simulink model "pipelined_and_spatial_parallelism"  (R2015b)
settings: Solver=FixedStepDiscrete  SolverMode=SingleTasking  StartTime=0.0  StopTime=5e-4  RelTol=1e-3
undefined symbols (not defined in the file): a, b
libraries: shlslibv1 x5277
(part 19 of 23)

== system pipelined_and_spatial_parallelism/Simon_encrypt 3/Key_expansion_function2 ==
  k_ii : Inport
  k_ii1 : Inport  Port=2
  k_ii2 : Inport  Port=3
  k_ii3 : Inport  Port=4
  c : Inport  Port=5
  z : Inport  Port=6
  Binary Logic{1..5} (5 alike) : shlslibv1/Math Functions/Binary Logic  syn_binlog_exp=a^b  synBlockType=primitive  synLatency=0  synBlockId=13
  Binary Logic6 : shlslibv1/Math Functions/Binary Logic  syn_binlog_exp=a|b  synBlockType=primitive  synLatency=0  synBlockId=13
  Binary Logic7 : shlslibv1/Math Functions/Binary Logic  syn_binlog_exp=a|b  synBlockType=primitive  synLatency=0  synBlockId=13
  Constant : shlslibv1/Sources/Constant  syn_cst_val=3  syn_cst_format=Specify  syn_cst_wl=4  syn_cst_fl=0  syn_cst_dt=unsigned  syn_cst_rnd=on  syn_cst_st=-1  synBlockType=primitive  synLatency=0  synBlockId=15
  Constant1 : shlslibv1/Sources/Constant  syn_cst_val=1  syn_cst_format=Specify  syn_cst_wl=4  syn_cst_fl=0  syn_cst_dt=unsigned  syn_cst_rnd=on  syn_cst_st=-1  synBlockType=primitive  synLatency=0  synBlockId=15
  Constant2 : shlslibv1/Sources/Constant  syn_cst_val=13  syn_cst_format=Specify  syn_cst_wl=4  syn_cst_fl=0  syn_cst_dt=unsigned  syn_cst_rnd=on  syn_cst_st=-1  synBlockType=primitive  synLatency=0  synBlockId=15
  Constant3 : shlslibv1/Sources/Constant  syn_cst_val=15  syn_cst_format=Specify  syn_cst_wl=4  syn_cst_fl=0  syn_cst_dt=unsigned  syn_cst_rnd=on  syn_cst_st=-1  synBlockType=primitive  synLatency=0  synBlockId=15
  Shifter : shlslibv1/Math Functions/Shifter  syn_shifter_opr=<<  syn_out_f=Automatic  syn_out_wl=16  syn_out_fl=8  syn_out_dt=signed  synBlockType=primitive  synLatency=0  synBlockId=12
  Shifter1 : shlslibv1/Math Functions/Shifter  syn_shifter_opr=>>  syn_out_f=Automatic  syn_out_wl=16  syn_out_fl=8  syn_out_dt=signed  synBlockType=primitive  synLatency=0  synBlockId=12
  Shifter2 : shlslibv1/Math Functions/Shifter  syn_shifter_opr=>>  syn_out_f=Automatic  syn_out_wl=16  syn_out_fl=8  syn_out_dt=signed  synBlockType=primitive  synLatency=0  synBlockId=12
  Shifter3 : shlslibv1/Math Functions/Shifter  syn_shifter_opr=<<  syn_out_f=Automatic  syn_out_wl=16  syn_out_fl=8  syn_out_dt=signed  synBlockType=primitive  synLatency=0  synBlockId=12
  K_iii : Outport
  Kiii1 : Outport  Port=2
  Kiii2 : Outport  Port=3
  Kiii3 : Outport  Port=4
  wires:
  Binary Logic1/1 -> Shifter3/1, Shifter2/1, Binary Logic3/2
  Constant/1 -> Shifter1/2
  Constant1/1 -> Shifter2/2
  Binary Logic2/1 -> Kiii3/1
  Binary Logic4/1 -> Binary Logic2/1
  k_ii/1 -> Binary Logic3/1
  k_ii1/1 -> K_iii/1, Binary Logic1/1
  z/1 -> Binary Logic5/1
  c/1 -> Binary Logic5/2
  k_ii2/1 -> Kiii1/1
  k_ii3/1 -> Shifter/1, Shifter1/1, Kiii2/1
  Binary Logic3/1 -> Binary Logic4/1
  Binary Logic5/1 -> Binary Logic2/2
  Constant2/1 -> Shifter/2
  Shifter1/1 -> Binary Logic6/1
  Shifter/1 -> Binary Logic6/2
  Binary Logic6/1 -> Binary Logic1/2
  Constant3/1 -> Shifter3/2
  Shifter2/1 -> Binary Logic7/1
  Shifter3/1 -> Binary Logic7/2
  Binary Logic7/1 -> Binary Logic4/2

== system pipelined_and_spatial_parallelism/Simon_encrypt 3/Key_expansion_function20 ==
  k_ii : Inport
  k_ii1 : Inport  Port=2
  k_ii2 : Inport  Port=3
  k_ii3 : Inport  Port=4
  c : Inport  Port=5
  z : Inport  Port=6
  Binary Logic{1..5} (5 alike) : shlslibv1/Math Functions/Binary Logic  syn_binlog_exp=a^b  synBlockType=primitive  synLatency=0  synBlockId=13
  Binary Logic6 : shlslibv1/Math Functions/Binary Logic  syn_binlog_exp=a|b  synBlockType=primitive  synLatency=0  synBlockId=13
  Binary Logic7 : shlslibv1/Math Functions/Binary Logic  syn_binlog_exp=a|b  synBlockType=primitive  synLatency=0  synBlockId=13
  Constant : shlslibv1/Sources/Constant  syn_cst_val=3  syn_cst_format=Specify  syn_cst_wl=4  syn_cst_fl=0  syn_cst_dt=unsigned  syn_cst_rnd=on  syn_cst_st=-1  synBlockType=primitive  synLatency=0  synBlockId=15
  Constant1 : shlslibv1/Sources/Constant  syn_cst_val=1  syn_cst_format=Specify  syn_cst_wl=4  syn_cst_fl=0  syn_cst_dt=unsigned  syn_cst_rnd=on  syn_cst_st=-1  synBlockType=primitive  synLatency=0  synBlockId=15
  Constant2 : shlslibv1/Sources/Constant  syn_cst_val=13  syn_cst_format=Specify  syn_cst_wl=4  syn_cst_fl=0  syn_cst_dt=unsigned  syn_cst_rnd=on  syn_cst_st=-1  synBlockType=primitive  synLatency=0  synBlockId=15
  Constant3 : shlslibv1/Sources/Constant  syn_cst_val=15  syn_cst_format=Specify  syn_cst_wl=4  syn_cst_fl=0  syn_cst_dt=unsigned  syn_cst_rnd=on  syn_cst_st=-1  synBlockType=primitive  synLatency=0  synBlockId=15
  Shifter : shlslibv1/Math Functions/Shifter  syn_shifter_opr=<<  syn_out_f=Automatic  syn_out_wl=16  syn_out_fl=8  syn_out_dt=signed  synBlockType=primitive  synLatency=0  synBlockId=12
  Shifter1 : shlslibv1/Math Functions/Shifter  syn_shifter_opr=>>  syn_out_f=Automatic  syn_out_wl=16  syn_out_fl=8  syn_out_dt=signed  synBlockType=primitive  synLatency=0  synBlockId=12
  Shifter2 : shlslibv1/Math Functions/Shifter  syn_shifter_opr=>>  syn_out_f=Automatic  syn_out_wl=16  syn_out_fl=8  syn_out_dt=signed  synBlockType=primitive  synLatency=0  synBlockId=12
  Shifter3 : shlslibv1/Math Functions/Shifter  syn_shifter_opr=<<  syn_out_f=Automatic  syn_out_wl=16  syn_out_fl=8  syn_out_dt=signed  synBlockType=primitive  synLatency=0  synBlockId=12
  K_iii : Outport
  Kiii1 : Outport  Port=2
  Kiii2 : Outport  Port=3
  Kiii3 : Outport  Port=4
  wires:
  Binary Logic1/1 -> Shifter3/1, Shifter2/1, Binary Logic3/2
  Constant/1 -> Shifter1/2
  Constant1/1 -> Shifter2/2
  Binary Logic2/1 -> Kiii3/1
  Binary Logic4/1 -> Binary Logic2/1
  k_ii/1 -> Binary Logic3/1
  k_ii1/1 -> K_iii/1, Binary Logic1/1
  z/1 -> Binary Logic5/1
  c/1 -> Binary Logic5/2
  k_ii2/1 -> Kiii1/1
  k_ii3/1 -> Shifter/1, Shifter1/1, Kiii2/1
  Binary Logic3/1 -> Binary Logic4/1
  Binary Logic5/1 -> Binary Logic2/2
  Constant2/1 -> Shifter/2
  Shifter1/1 -> Binary Logic6/1
  Shifter/1 -> Binary Logic6/2
  Binary Logic6/1 -> Binary Logic1/2
  Constant3/1 -> Shifter3/2
  Shifter2/1 -> Binary Logic7/1
  Shifter3/1 -> Binary Logic7/2
  Binary Logic7/1 -> Binary Logic4/2

== system pipelined_and_spatial_parallelism/Simon_encrypt 3/Key_expansion_function21 ==
  k_ii : Inport
  k_ii1 : Inport  Port=2
  k_ii2 : Inport  Port=3
  k_ii3 : Inport  Port=4
  c : Inport  Port=5
  z : Inport  Port=6
  Binary Logic{1..5} (5 alike) : shlslibv1/Math Functions/Binary Logic  syn_binlog_exp=a^b  synBlockType=primitive  synLatency=0  synBlockId=13
  Binary Logic6 : shlslibv1/Math Functions/Binary Logic  syn_binlog_exp=a|b  synBlockType=primitive  synLatency=0  synBlockId=13
  Binary Logic7 : shlslibv1/Math Functions/Binary Logic  syn_binlog_exp=a|b  synBlockType=primitive  synLatency=0  synBlockId=13
  Constant : shlslibv1/Sources/Constant  syn_cst_val=3  syn_cst_format=Specify  syn_cst_wl=4  syn_cst_fl=0  syn_cst_dt=unsigned  syn_cst_rnd=on  syn_cst_st=-1  synBlockType=primitive  synLatency=0  synBlockId=15
  Constant1 : shlslibv1/Sources/Constant  syn_cst_val=1  syn_cst_format=Specify  syn_cst_wl=4  syn_cst_fl=0  syn_cst_dt=unsigned  syn_cst_rnd=on  syn_cst_st=-1  synBlockType=primitive  synLatency=0  synBlockId=15
  Constant2 : shlslibv1/Sources/Constant  syn_cst_val=13  syn_cst_format=Specify  syn_cst_wl=4  syn_cst_fl=0  syn_cst_dt=unsigned  syn_cst_rnd=on  syn_cst_st=-1  synBlockType=primitive  synLatency=0  synBlockId=15
  Constant3 : shlslibv1/Sources/Constant  syn_cst_val=15  syn_cst_format=Specify  syn_cst_wl=4  syn_cst_fl=0  syn_cst_dt=unsigned  syn_cst_rnd=on  syn_cst_st=-1  synBlockType=primitive  synLatency=0  synBlockId=15
  Shifter : shlslibv1/Math Functions/Shifter  syn_shifter_opr=<<  syn_out_f=Automatic  syn_out_wl=16  syn_out_fl=8  syn_out_dt=signed  synBlockType=primitive  synLatency=0  synBlockId=12
  Shifter1 : shlslibv1/Math Functions/Shifter  syn_shifter_opr=>>  syn_out_f=Automatic  syn_out_wl=16  syn_out_fl=8  syn_out_dt=signed  synBlockType=primitive  synLatency=0  synBlockId=12
  Shifter2 : shlslibv1/Math Functions/Shifter  syn_shifter_opr=>>  syn_out_f=Automatic  syn_out_wl=16  syn_out_fl=8  syn_out_dt=signed  synBlockType=primitive  synLatency=0  synBlockId=12
  Shifter3 : shlslibv1/Math Functions/Shifter  syn_shifter_opr=<<  syn_out_f=Automatic  syn_out_wl=16  syn_out_fl=8  syn_out_dt=signed  synBlockType=primitive  synLatency=0  synBlockId=12
  K_iii : Outport
  Kiii1 : Outport  Port=2
  Kiii2 : Outport  Port=3
  Kiii3 : Outport  Port=4
  wires:
  Binary Logic1/1 -> Shifter3/1, Shifter2/1, Binary Logic3/2
  Constant/1 -> Shifter1/2
  Constant1/1 -> Shifter2/2
  Binary Logic2/1 -> Kiii3/1
  Binary Logic4/1 -> Binary Logic2/1
  k_ii/1 -> Binary Logic3/1
  k_ii1/1 -> K_iii/1, Binary Logic1/1
  z/1 -> Binary Logic5/1
  c/1 -> Binary Logic5/2
  k_ii2/1 -> Kiii1/1
  k_ii3/1 -> Shifter/1, Shifter1/1, Kiii2/1
  Binary Logic3/1 -> Binary Logic4/1
  Binary Logic5/1 -> Binary Logic2/2
  Constant2/1 -> Shifter/2
  Shifter1/1 -> Binary Logic6/1
  Shifter/1 -> Binary Logic6/2
  Binary Logic6/1 -> Binary Logic1/2
  Constant3/1 -> Shifter3/2
  Shifter2/1 -> Binary Logic7/1
  Shifter3/1 -> Binary Logic7/2
  Binary Logic7/1 -> Binary Logic4/2

== system pipelined_and_spatial_parallelism/Simon_encrypt 3/Key_expansion_function22 ==
  k_ii : Inport
  k_ii1 : Inport  Port=2
  k_ii2 : Inport  Port=3
  k_ii3 : Inport  Port=4
  c : Inport  Port=5
  z : Inport  Port=6
  Binary Logic{1..5} (5 alike) : shlslibv1/Math Functions/Binary Logic  syn_binlog_exp=a^b  synBlockType=primitive  synLatency=0  synBlockId=13
  Binary Logic6 : shlslibv1/Math Functions/Binary Logic  syn_binlog_exp=a|b  synBlockType=primitive  synLatency=0  synBlockId=13
  Binary Logic7 : shlslibv1/Math Functions/Binary Logic  syn_binlog_exp=a|b  synBlockType=primitive  synLatency=0  synBlockId=13
  Constant : shlslibv1/Sources/Constant  syn_cst_val=3  syn_cst_format=Specify  syn_cst_wl=4  syn_cst_fl=0  syn_cst_dt=unsigned  syn_cst_rnd=on  syn_cst_st=-1  synBlockType=primitive  synLatency=0  synBlockId=15
  Constant1 : shlslibv1/Sources/Constant  syn_cst_val=1  syn_cst_format=Specify  syn_cst_wl=4  syn_cst_fl=0  syn_cst_dt=unsigned  syn_cst_rnd=on  syn_cst_st=-1  synBlockType=primitive  synLatency=0  synBlockId=15
  Constant2 : shlslibv1/Sources/Constant  syn_cst_val=13  syn_cst_format=Specify  syn_cst_wl=4  syn_cst_fl=0  syn_cst_dt=unsigned  syn_cst_rnd=on  syn_cst_st=-1  synBlockType=primitive  synLatency=0  synBlockId=15
  Constant3 : shlslibv1/Sources/Constant  syn_cst_val=15  syn_cst_format=Specify  syn_cst_wl=4  syn_cst_fl=0  syn_cst_dt=unsigned  syn_cst_rnd=on  syn_cst_st=-1  synBlockType=primitive  synLatency=0  synBlockId=15
  Shifter : shlslibv1/Math Functions/Shifter  syn_shifter_opr=<<  syn_out_f=Automatic  syn_out_wl=16  syn_out_fl=8  syn_out_dt=signed  synBlockType=primitive  synLatency=0  synBlockId=12
  Shifter1 : shlslibv1/Math Functions/Shifter  syn_shifter_opr=>>  syn_out_f=Automatic  syn_out_wl=16  syn_out_fl=8  syn_out_dt=signed  synBlockType=primitive  synLatency=0  synBlockId=12
  Shifter2 : shlslibv1/Math Functions/Shifter  syn_shifter_opr=>>  syn_out_f=Automatic  syn_out_wl=16  syn_out_fl=8  syn_out_dt=signed  synBlockType=primitive  synLatency=0  synBlockId=12
  Shifter3 : shlslibv1/Math Functions/Shifter  syn_shifter_opr=<<  syn_out_f=Automatic  syn_out_wl=16  syn_out_fl=8  syn_out_dt=signed  synBlockType=primitive  synLatency=0  synBlockId=12
  K_iii : Outport
  Kiii1 : Outport  Port=2
  Kiii2 : Outport  Port=3
  Kiii3 : Outport  Port=4
  wires:
  Binary Logic1/1 -> Shifter3/1, Shifter2/1, Binary Logic3/2
  Constant/1 -> Shifter1/2
  Constant1/1 -> Shifter2/2
  Binary Logic2/1 -> Kiii3/1
  Binary Logic4/1 -> Binary Logic2/1
  k_ii/1 -> Binary Logic3/1
  k_ii1/1 -> K_iii/1, Binary Logic1/1
  z/1 -> Binary Logic5/1
  c/1 -> Binary Logic5/2
  k_ii2/1 -> Kiii1/1
  k_ii3/1 -> Shifter/1, Shifter1/1, Kiii2/1
  Binary Logic3/1 -> Binary Logic4/1
  Binary Logic5/1 -> Binary Logic2/2
  Constant2/1 -> Shifter/2
  Shifter1/1 -> Binary Logic6/1
  Shifter/1 -> Binary Logic6/2
  Binary Logic6/1 -> Binary Logic1/2
  Constant3/1 -> Shifter3/2
  Shifter2/1 -> Binary Logic7/1
  Shifter3/1 -> Binary Logic7/2
  Binary Logic7/1 -> Binary Logic4/2

== system pipelined_and_spatial_parallelism/Simon_encrypt 3/Key_expansion_function23 ==
  k_ii : Inport
  k_ii1 : Inport  Port=2
  k_ii2 : Inport  Port=3
  k_ii3 : Inport  Port=4
  c : Inport  Port=5
  z : Inport  Port=6
  Binary Logic{1..5} (5 alike) : shlslibv1/Math Functions/Binary Logic  syn_binlog_exp=a^b  synBlockType=primitive  synLatency=0  synBlockId=13
  Binary Logic6 : shlslibv1/Math Functions/Binary Logic  syn_binlog_exp=a|b  synBlockType=primitive  synLatency=0  synBlockId=13
  Binary Logic7 : shlslibv1/Math Functions/Binary Logic  syn_binlog_exp=a|b  synBlockType=primitive  synLatency=0  synBlockId=13
  Constant : shlslibv1/Sources/Constant  syn_cst_val=3  syn_cst_format=Specify  syn_cst_wl=4  syn_cst_fl=0  syn_cst_dt=unsigned  syn_cst_rnd=on  syn_cst_st=-1  synBlockType=primitive  synLatency=0  synBlockId=15
  Constant1 : shlslibv1/Sources/Constant  syn_cst_val=1  syn_cst_format=Specify  syn_cst_wl=4  syn_cst_fl=0  syn_cst_dt=unsigned  syn_cst_rnd=on  syn_cst_st=-1  synBlockType=primitive  synLatency=0  synBlockId=15
  Constant2 : shlslibv1/Sources/Constant  syn_cst_val=13  syn_cst_format=Specify  syn_cst_wl=4  syn_cst_fl=0  syn_cst_dt=unsigned  syn_cst_rnd=on  syn_cst_st=-1  synBlockType=primitive  synLatency=0  synBlockId=15
  Constant3 : shlslibv1/Sources/Constant  syn_cst_val=15  syn_cst_format=Specify  syn_cst_wl=4  syn_cst_fl=0  syn_cst_dt=unsigned  syn_cst_rnd=on  syn_cst_st=-1  synBlockType=primitive  synLatency=0  synBlockId=15
  Shifter : shlslibv1/Math Functions/Shifter  syn_shifter_opr=<<  syn_out_f=Automatic  syn_out_wl=16  syn_out_fl=8  syn_out_dt=signed  synBlockType=primitive  synLatency=0  synBlockId=12
  Shifter1 : shlslibv1/Math Functions/Shifter  syn_shifter_opr=>>  syn_out_f=Automatic  syn_out_wl=16  syn_out_fl=8  syn_out_dt=signed  synBlockType=primitive  synLatency=0  synBlockId=12
  Shifter2 : shlslibv1/Math Functions/Shifter  syn_shifter_opr=>>  syn_out_f=Automatic  syn_out_wl=16  syn_out_fl=8  syn_out_dt=signed  synBlockType=primitive  synLatency=0  synBlockId=12
  Shifter3 : shlslibv1/Math Functions/Shifter  syn_shifter_opr=<<  syn_out_f=Automatic  syn_out_wl=16  syn_out_fl=8  syn_out_dt=signed  synBlockType=primitive  synLatency=0  synBlockId=12
  K_iii : Outport
  Kiii1 : Outport  Port=2
  Kiii2 : Outport  Port=3
  Kiii3 : Outport  Port=4
  wires:
  Binary Logic1/1 -> Shifter3/1, Shifter2/1, Binary Logic3/2
  Constant/1 -> Shifter1/2
  Constant1/1 -> Shifter2/2
  Binary Logic2/1 -> Kiii3/1
  Binary Logic4/1 -> Binary Logic2/1
  k_ii/1 -> Binary Logic3/1
  k_ii1/1 -> K_iii/1, Binary Logic1/1
  z/1 -> Binary Logic5/1
  c/1 -> Binary Logic5/2
  k_ii2/1 -> Kiii1/1
  k_ii3/1 -> Shifter/1, Shifter1/1, Kiii2/1
  Binary Logic3/1 -> Binary Logic4/1
  Binary Logic5/1 -> Binary Logic2/2
  Constant2/1 -> Shifter/2
  Shifter1/1 -> Binary Logic6/1
  Shifter/1 -> Binary Logic6/2
  Binary Logic6/1 -> Binary Logic1/2
  Constant3/1 -> Shifter3/2
  Shifter2/1 -> Binary Logic7/1
  Shifter3/1 -> Binary Logic7/2
  Binary Logic7/1 -> Binary Logic4/2

== system pipelined_and_spatial_parallelism/Simon_encrypt 3/Key_expansion_function24 ==
  k_ii : Inport
  k_ii1 : Inport  Port=2
  k_ii2 : Inport  Port=3
  k_ii3 : Inport  Port=4
  c : Inport  Port=5
  z : Inport  Port=6
  Binary Logic{1..5} (5 alike) : shlslibv1/Math Functions/Binary Logic  syn_binlog_exp=a^b  synBlockType=primitive  synLatency=0  synBlockId=13
  Binary Logic6 : shlslibv1/Math Functions/Binary Logic  syn_binlog_exp=a|b  synBlockType=primitive  synLatency=0  synBlockId=13
  Binary Logic7 : shlslibv1/Math Functions/Binary Logic  syn_binlog_exp=a|b  synBlockType=primitive  synLatency=0  synBlockId=13
  Constant : shlslibv1/Sources/Constant  syn_cst_val=3  syn_cst_format=Specify  syn_cst_wl=4  syn_cst_fl=0  syn_cst_dt=unsigned  syn_cst_rnd=on  syn_cst_st=-1  synBlockType=primitive  synLatency=0  synBlockId=15
  Constant1 : shlslibv1/Sources/Constant  syn_cst_val=1  syn_cst_format=Specify  syn_cst_wl=4  syn_cst_fl=0  syn_cst_dt=unsigned  syn_cst_rnd=on  syn_cst_st=-1  synBlockType=primitive  synLatency=0  synBlockId=15
  Constant2 : shlslibv1/Sources/Constant  syn_cst_val=13  syn_cst_format=Specify  syn_cst_wl=4  syn_cst_fl=0  syn_cst_dt=unsigned  syn_cst_rnd=on  syn_cst_st=-1  synBlockType=primitive  synLatency=0  synBlockId=15
  Constant3 : shlslibv1/Sources/Constant  syn_cst_val=15  syn_cst_format=Specify  syn_cst_wl=4  syn_cst_fl=0  syn_cst_dt=unsigned  syn_cst_rnd=on  syn_cst_st=-1  synBlockType=primitive  synLatency=0  synBlockId=15
  Shifter : shlslibv1/Math Functions/Shifter  syn_shifter_opr=<<  syn_out_f=Automatic  syn_out_wl=16  syn_out_fl=8  syn_out_dt=signed  synBlockType=primitive  synLatency=0  synBlockId=12
  Shifter1 : shlslibv1/Math Functions/Shifter  syn_shifter_opr=>>  syn_out_f=Automatic  syn_out_wl=16  syn_out_fl=8  syn_out_dt=signed  synBlockType=primitive  synLatency=0  synBlockId=12
  Shifter2 : shlslibv1/Math Functions/Shifter  syn_shifter_opr=>>  syn_out_f=Automatic  syn_out_wl=16  syn_out_fl=8  syn_out_dt=signed  synBlockType=primitive  synLatency=0  synBlockId=12
  Shifter3 : shlslibv1/Math Functions/Shifter  syn_shifter_opr=<<  syn_out_f=Automatic  syn_out_wl=16  syn_out_fl=8  syn_out_dt=signed  synBlockType=primitive  synLatency=0  synBlockId=12
  K_iii : Outport
  Kiii1 : Outport  Port=2
  Kiii2 : Outport  Port=3
  Kiii3 : Outport  Port=4
  wires:
  Binary Logic1/1 -> Shifter3/1, Shifter2/1, Binary Logic3/2
  Constant/1 -> Shifter1/2
  Constant1/1 -> Shifter2/2
  Binary Logic2/1 -> Kiii3/1
  Binary Logic4/1 -> Binary Logic2/1
  k_ii/1 -> Binary Logic3/1
  k_ii1/1 -> K_iii/1, Binary Logic1/1
  z/1 -> Binary Logic5/1
  c/1 -> Binary Logic5/2
  k_ii2/1 -> Kiii1/1
  k_ii3/1 -> Shifter/1, Shifter1/1, Kiii2/1
  Binary Logic3/1 -> Binary Logic4/1
  Binary Logic5/1 -> Binary Logic2/2
  Constant2/1 -> Shifter/2
  Shifter1/1 -> Binary Logic6/1
  Shifter/1 -> Binary Logic6/2
  Binary Logic6/1 -> Binary Logic1/2
  Constant3/1 -> Shifter3/2
  Shifter2/1 -> Binary Logic7/1
  Shifter3/1 -> Binary Logic7/2
  Binary Logic7/1 -> Binary Logic4/2

== system pipelined_and_spatial_parallelism/Simon_encrypt 3/Key_expansion_function25 ==
  k_ii : Inport
  k_ii1 : Inport  Port=2
  k_ii2 : Inport  Port=3
  k_ii3 : Inport  Port=4
  c : Inport  Port=5
  z : Inport  Port=6
  Binary Logic{1..5} (5 alike) : shlslibv1/Math Functions/Binary Logic  syn_binlog_exp=a^b  synBlockType=primitive  synLatency=0  synBlockId=13
  Binary Logic6 : shlslibv1/Math Functions/Binary Logic  syn_binlog_exp=a|b  synBlockType=primitive  synLatency=0  synBlockId=13
  Binary Logic7 : shlslibv1/Math Functions/Binary Logic  syn_binlog_exp=a|b  synBlockType=primitive  synLatency=0  synBlockId=13
  Constant : shlslibv1/Sources/Constant  syn_cst_val=3  syn_cst_format=Specify  syn_cst_wl=4  syn_cst_fl=0  syn_cst_dt=unsigned  syn_cst_rnd=on  syn_cst_st=-1  synBlockType=primitive  synLatency=0  synBlockId=15
  Constant1 : shlslibv1/Sources/Constant  syn_cst_val=1  syn_cst_format=Specify  syn_cst_wl=4  syn_cst_fl=0  syn_cst_dt=unsigned  syn_cst_rnd=on  syn_cst_st=-1  synBlockType=primitive  synLatency=0  synBlockId=15
  Constant2 : shlslibv1/Sources/Constant  syn_cst_val=13  syn_cst_format=Specify  syn_cst_wl=4  syn_cst_fl=0  syn_cst_dt=unsigned  syn_cst_rnd=on  syn_cst_st=-1  synBlockType=primitive  synLatency=0  synBlockId=15
  Constant3 : shlslibv1/Sources/Constant  syn_cst_val=15  syn_cst_format=Specify  syn_cst_wl=4  syn_cst_fl=0  syn_cst_dt=unsigned  syn_cst_rnd=on  syn_cst_st=-1  synBlockType=primitive  synLatency=0  synBlockId=15
  Shifter : shlslibv1/Math Functions/Shifter  syn_shifter_opr=<<  syn_out_f=Automatic  syn_out_wl=16  syn_out_fl=8  syn_out_dt=signed  synBlockType=primitive  synLatency=0  synBlockId=12
  Shifter1 : shlslibv1/Math Functions/Shifter  syn_shifter_opr=>>  syn_out_f=Automatic  syn_out_wl=16  syn_out_fl=8  syn_out_dt=signed  synBlockType=primitive  synLatency=0  synBlockId=12
  Shifter2 : shlslibv1/Math Functions/Shifter  syn_shifter_opr=>>  syn_out_f=Automatic  syn_out_wl=16  syn_out_fl=8  syn_out_dt=signed  synBlockType=primitive  synLatency=0  synBlockId=12
  Shifter3 : shlslibv1/Math Functions/Shifter  syn_shifter_opr=<<  syn_out_f=Automatic  syn_out_wl=16  syn_out_fl=8  syn_out_dt=signed  synBlockType=primitive  synLatency=0  synBlockId=12
  K_iii : Outport
  Kiii1 : Outport  Port=2
  Kiii2 : Outport  Port=3
  Kiii3 : Outport  Port=4
  wires:
  Binary Logic1/1 -> Shifter3/1, Shifter2/1, Binary Logic3/2
  Constant/1 -> Shifter1/2
  Constant1/1 -> Shifter2/2
  Binary Logic2/1 -> Kiii3/1
  Binary Logic4/1 -> Binary Logic2/1
  k_ii/1 -> Binary Logic3/1
  k_ii1/1 -> K_iii/1, Binary Logic1/1
  z/1 -> Binary Logic5/1
  c/1 -> Binary Logic5/2
  k_ii2/1 -> Kiii1/1
  k_ii3/1 -> Shifter/1, Shifter1/1, Kiii2/1
  Binary Logic3/1 -> Binary Logic4/1
  Binary Logic5/1 -> Binary Logic2/2
  Constant2/1 -> Shifter/2
  Shifter1/1 -> Binary Logic6/1
  Shifter/1 -> Binary Logic6/2
  Binary Logic6/1 -> Binary Logic1/2
  Constant3/1 -> Shifter3/2
  Shifter2/1 -> Binary Logic7/1
  Shifter3/1 -> Binary Logic7/2
  Binary Logic7/1 -> Binary Logic4/2

== system pipelined_and_spatial_parallelism/Simon_encrypt 3/Key_expansion_function26 ==
  k_ii : Inport
  k_ii1 : Inport  Port=2
  k_ii2 : Inport  Port=3
  k_ii3 : Inport  Port=4
  c : Inport  Port=5
  z : Inport  Port=6
  Binary Logic{1..5} (5 alike) : shlslibv1/Math Functions/Binary Logic  syn_binlog_exp=a^b  synBlockType=primitive  synLatency=0  synBlockId=13
  Binary Logic6 : shlslibv1/Math Functions/Binary Logic  syn_binlog_exp=a|b  synBlockType=primitive  synLatency=0  synBlockId=13
  Binary Logic7 : shlslibv1/Math Functions/Binary Logic  syn_binlog_exp=a|b  synBlockType=primitive  synLatency=0  synBlockId=13
  Constant : shlslibv1/Sources/Constant  syn_cst_val=3  syn_cst_format=Specify  syn_cst_wl=4  syn_cst_fl=0  syn_cst_dt=unsigned  syn_cst_rnd=on  syn_cst_st=-1  synBlockType=primitive  synLatency=0  synBlockId=15
  Constant1 : shlslibv1/Sources/Constant  syn_cst_val=1  syn_cst_format=Specify  syn_cst_wl=4  syn_cst_fl=0  syn_cst_dt=unsigned  syn_cst_rnd=on  syn_cst_st=-1  synBlockType=primitive  synLatency=0  synBlockId=15
  Constant2 : shlslibv1/Sources/Constant  syn_cst_val=13  syn_cst_format=Specify  syn_cst_wl=4  syn_cst_fl=0  syn_cst_dt=unsigned  syn_cst_rnd=on  syn_cst_st=-1  synBlockType=primitive  synLatency=0  synBlockId=15
  Constant3 : shlslibv1/Sources/Constant  syn_cst_val=15  syn_cst_format=Specify  syn_cst_wl=4  syn_cst_fl=0  syn_cst_dt=unsigned  syn_cst_rnd=on  syn_cst_st=-1  synBlockType=primitive  synLatency=0  synBlockId=15
  Shifter : shlslibv1/Math Functions/Shifter  syn_shifter_opr=<<  syn_out_f=Automatic  syn_out_wl=16  syn_out_fl=8  syn_out_dt=signed  synBlockType=primitive  synLatency=0  synBlockId=12
  Shifter1 : shlslibv1/Math Functions/Shifter  syn_shifter_opr=>>  syn_out_f=Automatic  syn_out_wl=16  syn_out_fl=8  syn_out_dt=signed  synBlockType=primitive  synLatency=0  synBlockId=12
  Shifter2 : shlslibv1/Math Functions/Shifter  syn_shifter_opr=>>  syn_out_f=Automatic  syn_out_wl=16  syn_out_fl=8  syn_out_dt=signed  synBlockType=primitive  synLatency=0  synBlockId=12
  Shifter3 : shlslibv1/Math Functions/Shifter  syn_shifter_opr=<<  syn_out_f=Automatic  syn_out_wl=16  syn_out_fl=8  syn_out_dt=signed  synBlockType=primitive  synLatency=0  synBlockId=12
  K_iii : Outport
  Kiii1 : Outport  Port=2
  Kiii2 : Outport  Port=3
  Kiii3 : Outport  Port=4
  wires:
  Binary Logic1/1 -> Shifter3/1, Shifter2/1, Binary Logic3/2
  Constant/1 -> Shifter1/2
  Constant1/1 -> Shifter2/2
  Binary Logic2/1 -> Kiii3/1
  Binary Logic4/1 -> Binary Logic2/1
  k_ii/1 -> Binary Logic3/1
  k_ii1/1 -> K_iii/1, Binary Logic1/1
  z/1 -> Binary Logic5/1
  c/1 -> Binary Logic5/2
  k_ii2/1 -> Kiii1/1
  k_ii3/1 -> Shifter/1, Shifter1/1, Kiii2/1
  Binary Logic3/1 -> Binary Logic4/1
  Binary Logic5/1 -> Binary Logic2/2
  Constant2/1 -> Shifter/2
  Shifter1/1 -> Binary Logic6/1
  Shifter/1 -> Binary Logic6/2
  Binary Logic6/1 -> Binary Logic1/2
  Constant3/1 -> Shifter3/2
  Shifter2/1 -> Binary Logic7/1
  Shifter3/1 -> Binary Logic7/2
  Binary Logic7/1 -> Binary Logic4/2

== system pipelined_and_spatial_parallelism/Simon_encrypt 3/Key_expansion_function27 ==
  k_ii : Inport
  k_ii1 : Inport  Port=2
  k_ii2 : Inport  Port=3
  k_ii3 : Inport  Port=4
  c : Inport  Port=5
  z : Inport  Port=6
  Binary Logic{1..5} (5 alike) : shlslibv1/Math Functions/Binary Logic  syn_binlog_exp=a^b  synBlockType=primitive  synLatency=0  synBlockId=13
  Binary Logic6 : shlslibv1/Math Functions/Binary Logic  syn_binlog_exp=a|b  synBlockType=primitive  synLatency=0  synBlockId=13
  Binary Logic7 : shlslibv1/Math Functions/Binary Logic  syn_binlog_exp=a|b  synBlockType=primitive  synLatency=0  synBlockId=13
  Constant : shlslibv1/Sources/Constant  syn_cst_val=3  syn_cst_format=Specify  syn_cst_wl=4  syn_cst_fl=0  syn_cst_dt=unsigned  syn_cst_rnd=on  syn_cst_st=-1  synBlockType=primitive  synLatency=0  synBlockId=15
  Constant1 : shlslibv1/Sources/Constant  syn_cst_val=1  syn_cst_format=Specify  syn_cst_wl=4  syn_cst_fl=0  syn_cst_dt=unsigned  syn_cst_rnd=on  syn_cst_st=-1  synBlockType=primitive  synLatency=0  synBlockId=15
  Constant2 : shlslibv1/Sources/Constant  syn_cst_val=13  syn_cst_format=Specify  syn_cst_wl=4  syn_cst_fl=0  syn_cst_dt=unsigned  syn_cst_rnd=on  syn_cst_st=-1  synBlockType=primitive  synLatency=0  synBlockId=15
  Constant3 : shlslibv1/Sources/Constant  syn_cst_val=15  syn_cst_format=Specify  syn_cst_wl=4  syn_cst_fl=0  syn_cst_dt=unsigned  syn_cst_rnd=on  syn_cst_st=-1  synBlockType=primitive  synLatency=0  synBlockId=15
  Shifter : shlslibv1/Math Functions/Shifter  syn_shifter_opr=<<  syn_out_f=Automatic  syn_out_wl=16  syn_out_fl=8  syn_out_dt=signed  synBlockType=primitive  synLatency=0  synBlockId=12
  Shifter1 : shlslibv1/Math Functions/Shifter  syn_shifter_opr=>>  syn_out_f=Automatic  syn_out_wl=16  syn_out_fl=8  syn_out_dt=signed  synBlockType=primitive  synLatency=0  synBlockId=12
  Shifter2 : shlslibv1/Math Functions/Shifter  syn_shifter_opr=>>  syn_out_f=Automatic  syn_out_wl=16  syn_out_fl=8  syn_out_dt=signed  synBlockType=primitive  synLatency=0  synBlockId=12
  Shifter3 : shlslibv1/Math Functions/Shifter  syn_shifter_opr=<<  syn_out_f=Automatic  syn_out_wl=16  syn_out_fl=8  syn_out_dt=signed  synBlockType=primitive  synLatency=0  synBlockId=12
  K_iii : Outport
  Kiii1 : Outport  Port=2
  Kiii2 : Outport  Port=3
  Kiii3 : Outport  Port=4
  wires:
  Binary Logic1/1 -> Shifter3/1, Shifter2/1, Binary Logic3/2
  Constant/1 -> Shifter1/2
  Constant1/1 -> Shifter2/2
  Binary Logic2/1 -> Kiii3/1
  Binary Logic4/1 -> Binary Logic2/1
  k_ii/1 -> Binary Logic3/1
  k_ii1/1 -> K_iii/1, Binary Logic1/1
  z/1 -> Binary Logic5/1
  c/1 -> Binary Logic5/2
  k_ii2/1 -> Kiii1/1
  k_ii3/1 -> Shifter/1, Shifter1/1, Kiii2/1
  Binary Logic3/1 -> Binary Logic4/1
  Binary Logic5/1 -> Binary Logic2/2
  Constant2/1 -> Shifter/2
  Shifter1/1 -> Binary Logic6/1
  Shifter/1 -> Binary Logic6/2
  Binary Logic6/1 -> Binary Logic1/2
  Constant3/1 -> Shifter3/2
  Shifter2/1 -> Binary Logic7/1
  Shifter3/1 -> Binary Logic7/2
  Binary Logic7/1 -> Binary Logic4/2

== system pipelined_and_spatial_parallelism/Simon_encrypt 3/Key_expansion_function29 ==
  k_ii : Inport
  k_ii1 : Inport  Port=2
  k_ii2 : Inport  Port=3
  k_ii3 : Inport  Port=4
  c : Inport  Port=5
  z : Inport  Port=6
  Binary Logic{1..5} (5 alike) : shlslibv1/Math Functions/Binary Logic  syn_binlog_exp=a^b  synBlockType=primitive  synLatency=0  synBlockId=13
  Binary Logic6 : shlslibv1/Math Functions/Binary Logic  syn_binlog_exp=a|b  synBlockType=primitive  synLatency=0  synBlockId=13
  Binary Logic7 : shlslibv1/Math Functions/Binary Logic  syn_binlog_exp=a|b  synBlockType=primitive  synLatency=0  synBlockId=13
  Constant : shlslibv1/Sources/Constant  syn_cst_val=3  syn_cst_format=Specify  syn_cst_wl=4  syn_cst_fl=0  syn_cst_dt=unsigned  syn_cst_rnd=on  syn_cst_st=-1  synBlockType=primitive  synLatency=0  synBlockId=15
  Constant1 : shlslibv1/Sources/Constant  syn_cst_val=1  syn_cst_format=Specify  syn_cst_wl=4  syn_cst_fl=0  syn_cst_dt=unsigned  syn_cst_rnd=on  syn_cst_st=-1  synBlockType=primitive  synLatency=0  synBlockId=15
  Constant2 : shlslibv1/Sources/Constant  syn_cst_val=13  syn_cst_format=Specify  syn_cst_wl=4  syn_cst_fl=0  syn_cst_dt=unsigned  syn_cst_rnd=on  syn_cst_st=-1  synBlockType=primitive  synLatency=0  synBlockId=15
  Constant3 : shlslibv1/Sources/Constant  syn_cst_val=15  syn_cst_format=Specify  syn_cst_wl=4  syn_cst_fl=0  syn_cst_dt=unsigned  syn_cst_rnd=on  syn_cst_st=-1  synBlockType=primitive  synLatency=0  synBlockId=15
  Shifter : shlslibv1/Math Functions/Shifter  syn_shifter_opr=<<  syn_out_f=Automatic  syn_out_wl=16  syn_out_fl=8  syn_out_dt=signed  synBlockType=primitive  synLatency=0  synBlockId=12
  Shifter1 : shlslibv1/Math Functions/Shifter  syn_shifter_opr=>>  syn_out_f=Automatic  syn_out_wl=16  syn_out_fl=8  syn_out_dt=signed  synBlockType=primitive  synLatency=0  synBlockId=12
  Shifter2 : shlslibv1/Math Functions/Shifter  syn_shifter_opr=>>  syn_out_f=Automatic  syn_out_wl=16  syn_out_fl=8  syn_out_dt=signed  synBlockType=primitive  synLatency=0  synBlockId=12
  Shifter3 : shlslibv1/Math Functions/Shifter  syn_shifter_opr=<<  syn_out_f=Automatic  syn_out_wl=16  syn_out_fl=8  syn_out_dt=signed  synBlockType=primitive  synLatency=0  synBlockId=12
  K_iii : Outport
  Kiii1 : Outport  Port=2
  Kiii2 : Outport  Port=3
  Kiii3 : Outport  Port=4
  wires:
  Binary Logic1/1 -> Shifter3/1, Shifter2/1, Binary Logic3/2
  Constant/1 -> Shifter1/2
  Constant1/1 -> Shifter2/2
  Binary Logic2/1 -> Kiii3/1
  Binary Logic4/1 -> Binary Logic2/1
  k_ii/1 -> Binary Logic3/1
  k_ii1/1 -> K_iii/1, Binary Logic1/1
  z/1 -> Binary Logic5/1
  c/1 -> Binary Logic5/2
  k_ii2/1 -> Kiii1/1
  k_ii3/1 -> Shifter/1, Shifter1/1, Kiii2/1
  Binary Logic3/1 -> Binary Logic4/1
  Binary Logic5/1 -> Binary Logic2/2
  Constant2/1 -> Shifter/2
  Shifter1/1 -> Binary Logic6/1
  Shifter/1 -> Binary Logic6/2
  Binary Logic6/1 -> Binary Logic1/2
  Constant3/1 -> Shifter3/2
  Shifter2/1 -> Binary Logic7/1
  Shifter3/1 -> Binary Logic7/2
  Binary Logic7/1 -> Binary Logic4/2

== system pipelined_and_spatial_parallelism/Simon_encrypt 3/Key_expansion_function3 ==
  k_ii : Inport
  k_ii1 : Inport  Port=2
  k_ii2 : Inport  Port=3
  k_ii3 : Inport  Port=4
  c : Inport  Port=5
  z : Inport  Port=6
  Binary Logic{1..5} (5 alike) : shlslibv1/Math Functions/Binary Logic  syn_binlog_exp=a^b  synBlockType=primitive  synLatency=0  synBlockId=13
  Binary Logic6 : shlslibv1/Math Functions/Binary Logic  syn_binlog_exp=a|b  synBlockType=primitive  synLatency=0  synBlockId=13
  Binary Logic7 : shlslibv1/Math Functions/Binary Logic  syn_binlog_exp=a|b  synBlockType=primitive  synLatency=0  synBlockId=13
  Constant : shlslibv1/Sources/Constant  syn_cst_val=3  syn_cst_format=Specify  syn_cst_wl=4  syn_cst_fl=0  syn_cst_dt=unsigned  syn_cst_rnd=on  syn_cst_st=-1  synBlockType=primitive  synLatency=0  synBlockId=15
  Constant1 : shlslibv1/Sources/Constant  syn_cst_val=1  syn_cst_format=Specify  syn_cst_wl=4  syn_cst_fl=0  syn_cst_dt=unsigned  syn_cst_rnd=on  syn_cst_st=-1  synBlockType=primitive  synLatency=0  synBlockId=15
  Constant2 : shlslibv1/Sources/Constant  syn_cst_val=13  syn_cst_format=Specify  syn_cst_wl=4  syn_cst_fl=0  syn_cst_dt=unsigned  syn_cst_rnd=on  syn_cst_st=-1  synBlockType=primitive  synLatency=0  synBlockId=15
  Constant3 : shlslibv1/Sources/Constant  syn_cst_val=15  syn_cst_format=Specify  syn_cst_wl=4  syn_cst_fl=0  syn_cst_dt=unsigned  syn_cst_rnd=on  syn_cst_st=-1  synBlockType=primitive  synLatency=0  synBlockId=15
  Shifter : shlslibv1/Math Functions/Shifter  syn_shifter_opr=<<  syn_out_f=Automatic  syn_out_wl=16  syn_out_fl=8  syn_out_dt=signed  synBlockType=primitive  synLatency=0  synBlockId=12
  Shifter1 : shlslibv1/Math Functions/Shifter  syn_shifter_opr=>>  syn_out_f=Automatic  syn_out_wl=16  syn_out_fl=8  syn_out_dt=signed  synBlockType=primitive  synLatency=0  synBlockId=12
  Shifter2 : shlslibv1/Math Functions/Shifter  syn_shifter_opr=>>  syn_out_f=Automatic  syn_out_wl=16  syn_out_fl=8  syn_out_dt=signed  synBlockType=primitive  synLatency=0  synBlockId=12
  Shifter3 : shlslibv1/Math Functions/Shifter  syn_shifter_opr=<<  syn_out_f=Automatic  syn_out_wl=16  syn_out_fl=8  syn_out_dt=signed  synBlockType=primitive  synLatency=0  synBlockId=12
  K_iii : Outport
  Kiii1 : Outport  Port=2
  Kiii2 : Outport  Port=3
  Kiii3 : Outport  Port=4
  wires:
  Binary Logic1/1 -> Shifter3/1, Shifter2/1, Binary Logic3/2
  Constant/1 -> Shifter1/2
  Constant1/1 -> Shifter2/2
  Binary Logic2/1 -> Kiii3/1
  Binary Logic4/1 -> Binary Logic2/1
  k_ii/1 -> Binary Logic3/1
  k_ii1/1 -> K_iii/1, Binary Logic1/1
  z/1 -> Binary Logic5/1
  c/1 -> Binary Logic5/2
  k_ii2/1 -> Kiii1/1
  k_ii3/1 -> Shifter/1, Shifter1/1, Kiii2/1
  Binary Logic3/1 -> Binary Logic4/1
  Binary Logic5/1 -> Binary Logic2/2
  Constant2/1 -> Shifter/2
  Shifter1/1 -> Binary Logic6/1
  Shifter/1 -> Binary Logic6/2
  Binary Logic6/1 -> Binary Logic1/2
  Constant3/1 -> Shifter3/2
  Shifter2/1 -> Binary Logic7/1
  Shifter3/1 -> Binary Logic7/2
  Binary Logic7/1 -> Binary Logic4/2

== system pipelined_and_spatial_parallelism/Simon_encrypt 3/Key_expansion_function30 ==
  k_ii : Inport
  k_ii1 : Inport  Port=2
  k_ii2 : Inport  Port=3
  k_ii3 : Inport  Port=4
  c : Inport  Port=5
  z : Inport  Port=6
  Binary Logic{1..5} (5 alike) : shlslibv1/Math Functions/Binary Logic  syn_binlog_exp=a^b  synBlockType=primitive  synLatency=0  synBlockId=13
  Binary Logic6 : shlslibv1/Math Functions/Binary Logic  syn_binlog_exp=a|b  synBlockType=primitive  synLatency=0  synBlockId=13
  Binary Logic7 : shlslibv1/Math Functions/Binary Logic  syn_binlog_exp=a|b  synBlockType=primitive  synLatency=0  synBlockId=13
  Constant : shlslibv1/Sources/Constant  syn_cst_val=3  syn_cst_format=Specify  syn_cst_wl=4  syn_cst_fl=0  syn_cst_dt=unsigned  syn_cst_rnd=on  syn_cst_st=-1  synBlockType=primitive  synLatency=0  synBlockId=15
  Constant1 : shlslibv1/Sources/Constant  syn_cst_val=1  syn_cst_format=Specify  syn_cst_wl=4  syn_cst_fl=0  syn_cst_dt=unsigned  syn_cst_rnd=on  syn_cst_st=-1  synBlockType=primitive  synLatency=0  synBlockId=15
  Constant2 : shlslibv1/Sources/Constant  syn_cst_val=13  syn_cst_format=Specify  syn_cst_wl=4  syn_cst_fl=0  syn_cst_dt=unsigned  syn_cst_rnd=on  syn_cst_st=-1  synBlockType=primitive  synLatency=0  synBlockId=15
  Constant3 : shlslibv1/Sources/Constant  syn_cst_val=15  syn_cst_format=Specify  syn_cst_wl=4  syn_cst_fl=0  syn_cst_dt=unsigned  syn_cst_rnd=on  syn_cst_st=-1  synBlockType=primitive  synLatency=0  synBlockId=15
  Shifter : shlslibv1/Math Functions/Shifter  syn_shifter_opr=<<  syn_out_f=Automatic  syn_out_wl=16  syn_out_fl=8  syn_out_dt=signed  synBlockType=primitive  synLatency=0  synBlockId=12
  Shifter1 : shlslibv1/Math Functions/Shifter  syn_shifter_opr=>>  syn_out_f=Automatic  syn_out_wl=16  syn_out_fl=8  syn_out_dt=signed  synBlockType=primitive  synLatency=0  synBlockId=12
  Shifter2 : shlslibv1/Math Functions/Shifter  syn_shifter_opr=>>  syn_out_f=Automatic  syn_out_wl=16  syn_out_fl=8  syn_out_dt=signed  synBlockType=primitive  synLatency=0  synBlockId=12
  Shifter3 : shlslibv1/Math Functions/Shifter  syn_shifter_opr=<<  syn_out_f=Automatic  syn_out_wl=16  syn_out_fl=8  syn_out_dt=signed  synBlockType=primitive  synLatency=0  synBlockId=12
  K_iii : Outport
  Kiii1 : Outport  Port=2
  Kiii2 : Outport  Port=3
  Kiii3 : Outport  Port=4
  wires:
  Binary Logic1/1 -> Shifter3/1, Shifter2/1, Binary Logic3/2
  Constant/1 -> Shifter1/2
  Constant1/1 -> Shifter2/2
  Binary Logic2/1 -> Kiii3/1
  Binary Logic4/1 -> Binary Logic2/1
  k_ii/1 -> Binary Logic3/1
  k_ii1/1 -> K_iii/1, Binary Logic1/1
  z/1 -> Binary Logic5/1
  c/1 -> Binary Logic5/2
  k_ii2/1 -> Kiii1/1
  k_ii3/1 -> Shifter/1, Shifter1/1, Kiii2/1
  Binary Logic3/1 -> Binary Logic4/1
  Binary Logic5/1 -> Binary Logic2/2
  Constant2/1 -> Shifter/2
  Shifter1/1 -> Binary Logic6/1
  Shifter/1 -> Binary Logic6/2
  Binary Logic6/1 -> Binary Logic1/2
  Constant3/1 -> Shifter3/2
  Shifter2/1 -> Binary Logic7/1
  Shifter3/1 -> Binary Logic7/2
  Binary Logic7/1 -> Binary Logic4/2

== system pipelined_and_spatial_parallelism/Simon_encrypt 3/Key_expansion_function31 ==
  k_ii : Inport
  k_ii1 : Inport  Port=2
  k_ii2 : Inport  Port=3
  k_ii3 : Inport  Port=4
  c : Inport  Port=5
  z : Inport  Port=6
  Binary Logic{1..5} (5 alike) : shlslibv1/Math Functions/Binary Logic  syn_binlog_exp=a^b  synBlockType=primitive  synLatency=0  synBlockId=13
  Binary Logic6 : shlslibv1/Math Functions/Binary Logic  syn_binlog_exp=a|b  synBlockType=primitive  synLatency=0  synBlockId=13
  Binary Logic7 : shlslibv1/Math Functions/Binary Logic  syn_binlog_exp=a|b  synBlockType=primitive  synLatency=0  synBlockId=13
  Constant : shlslibv1/Sources/Constant  syn_cst_val=3  syn_cst_format=Specify  syn_cst_wl=4  syn_cst_fl=0  syn_cst_dt=unsigned  syn_cst_rnd=on  syn_cst_st=-1  synBlockType=primitive  synLatency=0  synBlockId=15
  Constant1 : shlslibv1/Sources/Constant  syn_cst_val=1  syn_cst_format=Specify  syn_cst_wl=4  syn_cst_fl=0  syn_cst_dt=unsigned  syn_cst_rnd=on  syn_cst_st=-1  synBlockType=primitive  synLatency=0  synBlockId=15
  Constant2 : shlslibv1/Sources/Constant  syn_cst_val=13  syn_cst_format=Specify  syn_cst_wl=4  syn_cst_fl=0  syn_cst_dt=unsigned  syn_cst_rnd=on  syn_cst_st=-1  synBlockType=primitive  synLatency=0  synBlockId=15
  Constant3 : shlslibv1/Sources/Constant  syn_cst_val=15  syn_cst_format=Specify  syn_cst_wl=4  syn_cst_fl=0  syn_cst_dt=unsigned  syn_cst_rnd=on  syn_cst_st=-1  synBlockType=primitive  synLatency=0  synBlockId=15
  Shifter : shlslibv1/Math Functions/Shifter  syn_shifter_opr=<<  syn_out_f=Automatic  syn_out_wl=16  syn_out_fl=8  syn_out_dt=signed  synBlockType=primitive  synLatency=0  synBlockId=12
  Shifter1 : shlslibv1/Math Functions/Shifter  syn_shifter_opr=>>  syn_out_f=Automatic  syn_out_wl=16  syn_out_fl=8  syn_out_dt=signed  synBlockType=primitive  synLatency=0  synBlockId=12
  Shifter2 : shlslibv1/Math Functions/Shifter  syn_shifter_opr=>>  syn_out_f=Automatic  syn_out_wl=16  syn_out_fl=8  syn_out_dt=signed  synBlockType=primitive  synLatency=0  synBlockId=12
  Shifter3 : shlslibv1/Math Functions/Shifter  syn_shifter_opr=<<  syn_out_f=Automatic  syn_out_wl=16  syn_out_fl=8  syn_out_dt=signed  synBlockType=primitive  synLatency=0  synBlockId=12
  K_iii : Outport
  Kiii1 : Outport  Port=2
  Kiii2 : Outport  Port=3
  Kiii3 : Outport  Port=4
  wires:
  Binary Logic1/1 -> Shifter3/1, Shifter2/1, Binary Logic3/2
  Constant/1 -> Shifter1/2
  Constant1/1 -> Shifter2/2
  Binary Logic2/1 -> Kiii3/1
  Binary Logic4/1 -> Binary Logic2/1
  k_ii/1 -> Binary Logic3/1
  k_ii1/1 -> K_iii/1, Binary Logic1/1
  z/1 -> Binary Logic5/1
  c/1 -> Binary Logic5/2
  k_ii2/1 -> Kiii1/1
  k_ii3/1 -> Shifter/1, Shifter1/1, Kiii2/1
  Binary Logic3/1 -> Binary Logic4/1
  Binary Logic5/1 -> Binary Logic2/2
  Constant2/1 -> Shifter/2
  Shifter1/1 -> Binary Logic6/1
  Shifter/1 -> Binary Logic6/2
  Binary Logic6/1 -> Binary Logic1/2
  Constant3/1 -> Shifter3/2
  Shifter2/1 -> Binary Logic7/1
  Shifter3/1 -> Binary Logic7/2
  Binary Logic7/1 -> Binary Logic4/2

== system pipelined_and_spatial_parallelism/Simon_encrypt 3/Key_expansion_function32 ==
  k_ii : Inport
  k_ii1 : Inport  Port=2
  k_ii2 : Inport  Port=3
  k_ii3 : Inport  Port=4
  c : Inport  Port=5
  z : Inport  Port=6
  Binary Logic{1..5} (5 alike) : shlslibv1/Math Functions/Binary Logic  syn_binlog_exp=a^b  synBlockType=primitive  synLatency=0  synBlockId=13
  Binary Logic6 : shlslibv1/Math Functions/Binary Logic  syn_binlog_exp=a|b  synBlockType=primitive  synLatency=0  synBlockId=13
  Binary Logic7 : shlslibv1/Math Functions/Binary Logic  syn_binlog_exp=a|b  synBlockType=primitive  synLatency=0  synBlockId=13
  Constant : shlslibv1/Sources/Constant  syn_cst_val=3  syn_cst_format=Specify  syn_cst_wl=4  syn_cst_fl=0  syn_cst_dt=unsigned  syn_cst_rnd=on  syn_cst_st=-1  synBlockType=primitive  synLatency=0  synBlockId=15
  Constant1 : shlslibv1/Sources/Constant  syn_cst_val=1  syn_cst_format=Specify  syn_cst_wl=4  syn_cst_fl=0  syn_cst_dt=unsigned  syn_cst_rnd=on  syn_cst_st=-1  synBlockType=primitive  synLatency=0  synBlockId=15
  Constant2 : shlslibv1/Sources/Constant  syn_cst_val=13  syn_cst_format=Specify  syn_cst_wl=4  syn_cst_fl=0  syn_cst_dt=unsigned  syn_cst_rnd=on  syn_cst_st=-1  synBlockType=primitive  synLatency=0  synBlockId=15
  Constant3 : shlslibv1/Sources/Constant  syn_cst_val=15  syn_cst_format=Specify  syn_cst_wl=4  syn_cst_fl=0  syn_cst_dt=unsigned  syn_cst_rnd=on  syn_cst_st=-1  synBlockType=primitive  synLatency=0  synBlockId=15
  Shifter : shlslibv1/Math Functions/Shifter  syn_shifter_opr=<<  syn_out_f=Automatic  syn_out_wl=16  syn_out_fl=8  syn_out_dt=signed  synBlockType=primitive  synLatency=0  synBlockId=12
  Shifter1 : shlslibv1/Math Functions/Shifter  syn_shifter_opr=>>  syn_out_f=Automatic  syn_out_wl=16  syn_out_fl=8  syn_out_dt=signed  synBlockType=primitive  synLatency=0  synBlockId=12
  Shifter2 : shlslibv1/Math Functions/Shifter  syn_shifter_opr=>>  syn_out_f=Automatic  syn_out_wl=16  syn_out_fl=8  syn_out_dt=signed  synBlockType=primitive  synLatency=0  synBlockId=12
  Shifter3 : shlslibv1/Math Functions/Shifter  syn_shifter_opr=<<  syn_out_f=Automatic  syn_out_wl=16  syn_out_fl=8  syn_out_dt=signed  synBlockType=primitive  synLatency=0  synBlockId=12
  K_iii : Outport
  Kiii1 : Outport  Port=2
  Kiii2 : Outport  Port=3
  Kiii3 : Outport  Port=4
  wires:
  Binary Logic1/1 -> Shifter3/1, Shifter2/1, Binary Logic3/2
  Constant/1 -> Shifter1/2
  Constant1/1 -> Shifter2/2
  Binary Logic2/1 -> Kiii3/1
  Binary Logic4/1 -> Binary Logic2/1
  k_ii/1 -> Binary Logic3/1
  k_ii1/1 -> K_iii/1, Binary Logic1/1
  z/1 -> Binary Logic5/1
  c/1 -> Binary Logic5/2
  k_ii2/1 -> Kiii1/1
  k_ii3/1 -> Shifter/1, Shifter1/1, Kiii2/1
  Binary Logic3/1 -> Binary Logic4/1
  Binary Logic5/1 -> Binary Logic2/2
  Constant2/1 -> Shifter/2
  Shifter1/1 -> Binary Logic6/1
  Shifter/1 -> Binary Logic6/2
  Binary Logic6/1 -> Binary Logic1/2
  Constant3/1 -> Shifter3/2
  Shifter2/1 -> Binary Logic7/1
  Shifter3/1 -> Binary Logic7/2
  Binary Logic7/1 -> Binary Logic4/2

== system pipelined_and_spatial_parallelism/Simon_encrypt 3/Key_expansion_function4 ==
  k_ii : Inport
  k_ii1 : Inport  Port=2
  k_ii2 : Inport  Port=3
  k_ii3 : Inport  Port=4
  c : Inport  Port=5
  z : Inport  Port=6
  Binary Logic{1..5} (5 alike) : shlslibv1/Math Functions/Binary Logic  syn_binlog_exp=a^b  synBlockType=primitive  synLatency=0  synBlockId=13
  Binary Logic6 : shlslibv1/Math Functions/Binary Logic  syn_binlog_exp=a|b  synBlockType=primitive  synLatency=0  synBlockId=13
  Binary Logic7 : shlslibv1/Math Functions/Binary Logic  syn_binlog_exp=a|b  synBlockType=primitive  synLatency=0  synBlockId=13
  Constant : shlslibv1/Sources/Constant  syn_cst_val=3  syn_cst_format=Specify  syn_cst_wl=4  syn_cst_fl=0  syn_cst_dt=unsigned  syn_cst_rnd=on  syn_cst_st=-1  synBlockType=primitive  synLatency=0  synBlockId=15
  Constant1 : shlslibv1/Sources/Constant  syn_cst_val=1  syn_cst_format=Specify  syn_cst_wl=4  syn_cst_fl=0  syn_cst_dt=unsigned  syn_cst_rnd=on  syn_cst_st=-1  synBlockType=primitive  synLatency=0  synBlockId=15
  Constant2 : shlslibv1/Sources/Constant  syn_cst_val=13  syn_cst_format=Specify  syn_cst_wl=4  syn_cst_fl=0  syn_cst_dt=unsigned  syn_cst_rnd=on  syn_cst_st=-1  synBlockType=primitive  synLatency=0  synBlockId=15
  Constant3 : shlslibv1/Sources/Constant  syn_cst_val=15  syn_cst_format=Specify  syn_cst_wl=4  syn_cst_fl=0  syn_cst_dt=unsigned  syn_cst_rnd=on  syn_cst_st=-1  synBlockType=primitive  synLatency=0  synBlockId=15
  Shifter : shlslibv1/Math Functions/Shifter  syn_shifter_opr=<<  syn_out_f=Automatic  syn_out_wl=16  syn_out_fl=8  syn_out_dt=signed  synBlockType=primitive  synLatency=0  synBlockId=12
  Shifter1 : shlslibv1/Math Functions/Shifter  syn_shifter_opr=>>  syn_out_f=Automatic  syn_out_wl=16  syn_out_fl=8  syn_out_dt=signed  synBlockType=primitive  synLatency=0  synBlockId=12
  Shifter2 : shlslibv1/Math Functions/Shifter  syn_shifter_opr=>>  syn_out_f=Automatic  syn_out_wl=16  syn_out_fl=8  syn_out_dt=signed  synBlockType=primitive  synLatency=0  synBlockId=12
  Shifter3 : shlslibv1/Math Functions/Shifter  syn_shifter_opr=<<  syn_out_f=Automatic  syn_out_wl=16  syn_out_fl=8  syn_out_dt=signed  synBlockType=primitive  synLatency=0  synBlockId=12
  K_iii : Outport
  Kiii1 : Outport  Port=2
  Kiii2 : Outport  Port=3
  Kiii3 : Outport  Port=4
  wires:
  Binary Logic1/1 -> Shifter3/1, Shifter2/1, Binary Logic3/2
  Constant/1 -> Shifter1/2
  Constant1/1 -> Shifter2/2
  Binary Logic2/1 -> Kiii3/1
  Binary Logic4/1 -> Binary Logic2/1
  k_ii/1 -> Binary Logic3/1
  k_ii1/1 -> K_iii/1, Binary Logic1/1
  z/1 -> Binary Logic5/1
  c/1 -> Binary Logic5/2
  k_ii2/1 -> Kiii1/1
  k_ii3/1 -> Shifter/1, Shifter1/1, Kiii2/1
  Binary Logic3/1 -> Binary Logic4/1
  Binary Logic5/1 -> Binary Logic2/2
  Constant2/1 -> Shifter/2
  Shifter1/1 -> Binary Logic6/1
  Shifter/1 -> Binary Logic6/2
  Binary Logic6/1 -> Binary Logic1/2
  Constant3/1 -> Shifter3/2
  Shifter2/1 -> Binary Logic7/1
  Shifter3/1 -> Binary Logic7/2
  Binary Logic7/1 -> Binary Logic4/2

== system pipelined_and_spatial_parallelism/Simon_encrypt 3/Key_expansion_function5 ==
  k_ii : Inport
  k_ii1 : Inport  Port=2
  k_ii2 : Inport  Port=3
  k_ii3 : Inport  Port=4
  c : Inport  Port=5
  z : Inport  Port=6
  Binary Logic{1..5} (5 alike) : shlslibv1/Math Functions/Binary Logic  syn_binlog_exp=a^b  synBlockType=primitive  synLatency=0  synBlockId=13
  Binary Logic6 : shlslibv1/Math Functions/Binary Logic  syn_binlog_exp=a|b  synBlockType=primitive  synLatency=0  synBlockId=13
  Binary Logic7 : shlslibv1/Math Functions/Binary Logic  syn_binlog_exp=a|b  synBlockType=primitive  synLatency=0  synBlockId=13
  Constant : shlslibv1/Sources/Constant  syn_cst_val=3  syn_cst_format=Specify  syn_cst_wl=4  syn_cst_fl=0  syn_cst_dt=unsigned  syn_cst_rnd=on  syn_cst_st=-1  synBlockType=primitive  synLatency=0  synBlockId=15
  Constant1 : shlslibv1/Sources/Constant  syn_cst_val=1  syn_cst_format=Specify  syn_cst_wl=4  syn_cst_fl=0  syn_cst_dt=unsigned  syn_cst_rnd=on  syn_cst_st=-1  synBlockType=primitive  synLatency=0  synBlockId=15
  Constant2 : shlslibv1/Sources/Constant  syn_cst_val=13  syn_cst_format=Specify  syn_cst_wl=4  syn_cst_fl=0  syn_cst_dt=unsigned  syn_cst_rnd=on  syn_cst_st=-1  synBlockType=primitive  synLatency=0  synBlockId=15
  Constant3 : shlslibv1/Sources/Constant  syn_cst_val=15  syn_cst_format=Specify  syn_cst_wl=4  syn_cst_fl=0  syn_cst_dt=unsigned  syn_cst_rnd=on  syn_cst_st=-1  synBlockType=primitive  synLatency=0  synBlockId=15
  Shifter : shlslibv1/Math Functions/Shifter  syn_shifter_opr=<<  syn_out_f=Automatic  syn_out_wl=16  syn_out_fl=8  syn_out_dt=signed  synBlockType=primitive  synLatency=0  synBlockId=12
  Shifter1 : shlslibv1/Math Functions/Shifter  syn_shifter_opr=>>  syn_out_f=Automatic  syn_out_wl=16  syn_out_fl=8  syn_out_dt=signed  synBlockType=primitive  synLatency=0  synBlockId=12
  Shifter2 : shlslibv1/Math Functions/Shifter  syn_shifter_opr=>>  syn_out_f=Automatic  syn_out_wl=16  syn_out_fl=8  syn_out_dt=signed  synBlockType=primitive  synLatency=0  synBlockId=12
  Shifter3 : shlslibv1/Math Functions/Shifter  syn_shifter_opr=<<  syn_out_f=Automatic  syn_out_wl=16  syn_out_fl=8  syn_out_dt=signed  synBlockType=primitive  synLatency=0  synBlockId=12
  K_iii : Outport
  Kiii1 : Outport  Port=2
  Kiii2 : Outport  Port=3
  Kiii3 : Outport  Port=4
  wires:
  Binary Logic1/1 -> Shifter3/1, Shifter2/1, Binary Logic3/2
  Constant/1 -> Shifter1/2
  Constant1/1 -> Shifter2/2
  Binary Logic2/1 -> Kiii3/1
  Binary Logic4/1 -> Binary Logic2/1
  k_ii/1 -> Binary Logic3/1
  k_ii1/1 -> K_iii/1, Binary Logic1/1
  z/1 -> Binary Logic5/1
  c/1 -> Binary Logic5/2
  k_ii2/1 -> Kiii1/1
  k_ii3/1 -> Shifter/1, Shifter1/1, Kiii2/1
  Binary Logic3/1 -> Binary Logic4/1
  Binary Logic5/1 -> Binary Logic2/2
  Constant2/1 -> Shifter/2
  Shifter1/1 -> Binary Logic6/1
  Shifter/1 -> Binary Logic6/2
  Binary Logic6/1 -> Binary Logic1/2
  Constant3/1 -> Shifter3/2
  Shifter2/1 -> Binary Logic7/1
  Shifter3/1 -> Binary Logic7/2
  Binary Logic7/1 -> Binary Logic4/2
